simulink model "gm_counter"  (R2021b)
settings: Solver=VariableStepAuto  StartTime=0.0  StopTime=96e-06  RelTol=1e-3
libraries: simulink x1
settings Model: Creator=Marco Milanesi  LastModifiedBy=Marco Milanesi
settings OptimizationCC: BlockReduction=off  ConditionallyExecuteInputs=off
settings DebuggingCC: InheritedTsInSrcMsg=none

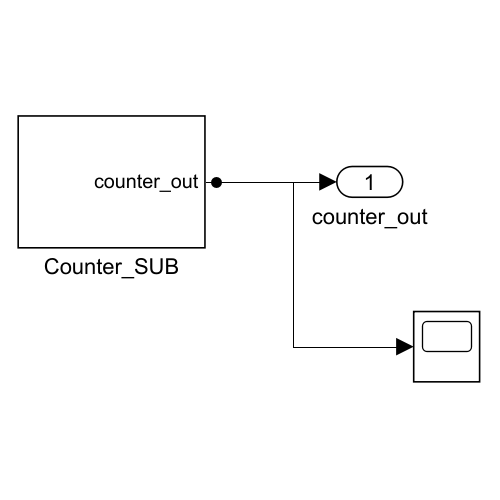
[thumbnail: Simulink's stored preview of the top-level diagram]
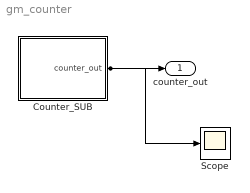
== system gm_counter ==
  Counter_SUB : Subsystem
  Scope : Scope
  counter_out : Outport
  wires:
  Counter_SUB/1(counter_out) -> counter_out/1, Scope/1

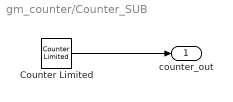
== system gm_counter/Counter_SUB ==
  Counter Limited : simulink/Sources/Counter Limited  uplimit=1024  tsamp=1e-03
  counter_out : Outport
  wires:
  Counter Limited/1 -> counter_out/1
